simulink model "SIMULINK_CHUA"  (R2022b)
settings: Solver=VariableStepAuto  StartTime=0.0  StopTime=200  RelTol=1e-3
values from neighbouring files (symbols this model uses):
  a = 15.6    [diode1.m]    (also in simulink_main.m)
  b = 28    [diode1.m]    (also in simulink_main.m)
  c = r0*R*c2/L    (= 0.283616666667)    [simulink_main.m]
  x0 = [0.7; 0; 0+ 1E-12]    [simulink_main.m]
settings Model: Creator=mluser  LastModifiedBy=mluser

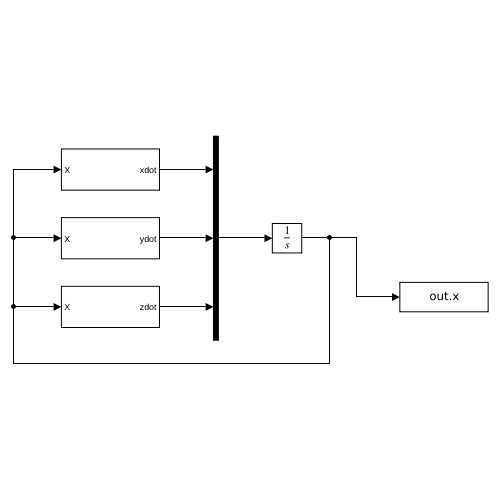
[thumbnail: Simulink's stored preview of the top-level diagram]
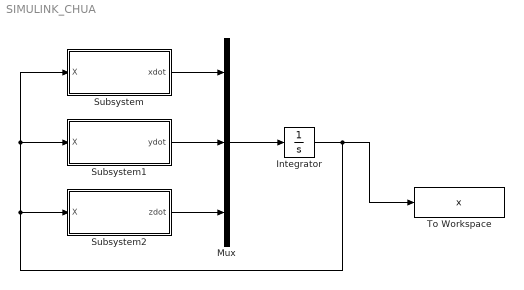
== system SIMULINK_CHUA ==
  Integrator : Integrator  InitialCondition=x0
  Mux : Mux  Inputs=3
  Subsystem : Subsystem
  Subsystem1 : Subsystem
  Subsystem2 : Subsystem
  To Workspace : ToWorkspace  VariableName=x  SaveFormat=Structure With Time  SampleTime=-1
  wires:
  Subsystem2/1(zdot) -> Mux/3
  Subsystem1/1(ydot) -> Mux/2
  Subsystem/1(xdot) -> Mux/1
  Mux/1 -> Integrator/1
  Integrator/1 -> To Workspace/1, Subsystem1/1(X), Subsystem/1(X), Subsystem2/1(X)

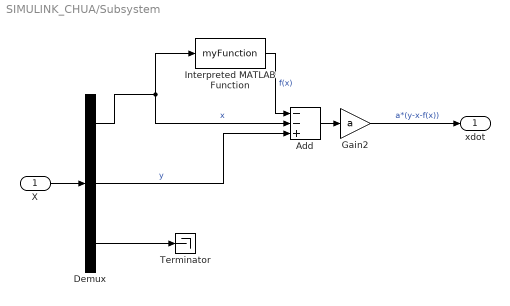
== system SIMULINK_CHUA/Subsystem ==
  X : Inport
  Add : Sum  Inputs=--+
  Demux : Demux  Outputs=3
  Gain2 : Gain  Gain=a
  Interpreted MATLAB Function : MATLABFcn  MATLABFcn=myFunction
  Terminator : Terminator
  xdot : Outport
  wires:
  X/1 -> Demux/1
  Demux/1 -> Add/2, Interpreted MATLAB Function/1  "x"
  Demux/2 -> Add/3  "y"
  Add/1 -> Gain2/1
  Demux/3 -> Terminator/1
  Interpreted MATLAB Function/1 -> Add/1  "f(x)"
  Gain2/1 -> xdot/1  "a*(y-x-f(x))"

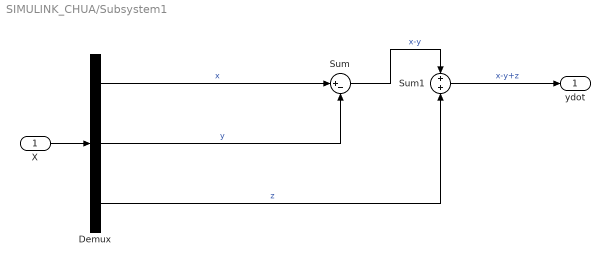
== system SIMULINK_CHUA/Subsystem1 ==
  X : Inport
  Demux : Demux  Outputs=3
  Sum : Sum  Inputs=|+-
  Sum1 : Sum
  ydot : Outport
  wires:
  Demux/1 -> Sum/1  "x"
  Demux/2 -> Sum/2  "y"
  X/1 -> Demux/1
  Demux/3 -> Sum1/2  "z"
  Sum/1 -> Sum1/1  "x-y"
  Sum1/1 -> ydot/1  "x-y+z"

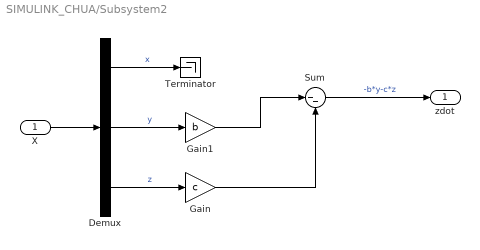
== system SIMULINK_CHUA/Subsystem2 ==
  X : Inport
  Demux : Demux  Outputs=3
  Gain : Gain  Gain=c
  Gain1 : Gain  Gain=b
  Sum : Sum  Inputs=|--
  Terminator : Terminator
  zdot : Outport
  wires:
  X/1 -> Demux/1
  Demux/1 -> Terminator/1  "x"
  Demux/2 -> Gain1/1  "y"
  Demux/3 -> Gain/1  "z"
  Gain1/1 -> Sum/1
  Gain/1 -> Sum/2
  Sum/1 -> zdot/1  "-b*y-c*z"
